simulink model "PistonDynamics"  (R2012b)
settings: Solver=ode45  StartTime=0.0  StopTime=5.0  RelTol=1e-3
undefined symbols (not defined in the file or in its folder): Ap, Ap_seal, Ar_seal, Bkp_seal, Bp1, frictionstribeck_velocity, Ka1, Lp_seal, Lr_seal, Mp1, seal_compression, seal_hardness, SealConstValue, SealType, Xp_init
settings Model: Creator=HBALLEST  LastModifiedBy=HBALLEST

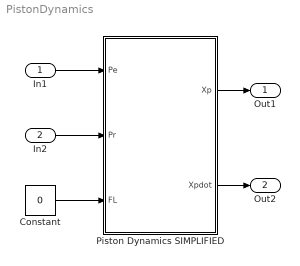
== system PistonDynamics ==
  In1 : Inport
  In2 : Inport  Port=2
  Constant : Constant  Value=0
  Piston Dynamics SIMPLIFIED : Subsystem
  Out1 : Outport
  Out2 : Outport  Port=2
  wires:
  Constant/1 -> Piston Dynamics SIMPLIFIED/3(FL)
  Piston Dynamics SIMPLIFIED/1(Xp) -> Out1/1
  Piston Dynamics SIMPLIFIED/2(Xpdot) -> Out2/1
  In2/1 -> Piston Dynamics SIMPLIFIED/2(Pr)
  In1/1 -> Piston Dynamics SIMPLIFIED/1(Pe)

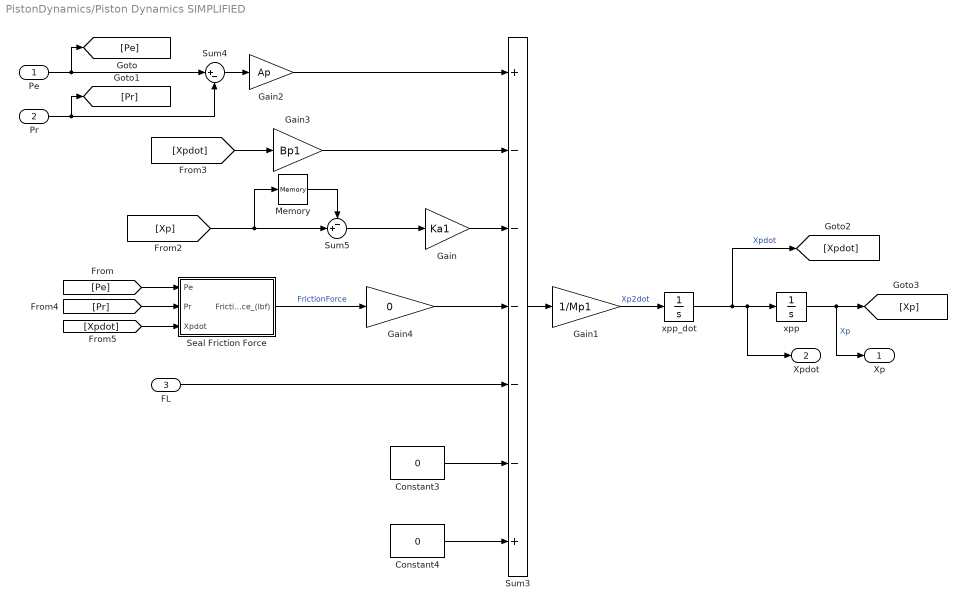
== system PistonDynamics/Piston Dynamics SIMPLIFIED ==
  Pe : Inport
  Pr : Inport  Port=2
  FL : Inport  Port=3
  Constant3 : Constant  Value=0
  Constant4 : Constant  Value=0
  Gain : Gain  Gain=Ka1
  Gain1 : Gain  Gain=1/Mp1
  Gain2 : Gain  Gain=Ap
  Gain3 : Gain  Gain=Bp1
  Gain4 : Gain  Gain=0
  Memory : Memory
  Seal Friction Force : Subsystem
  Sum3 : Sum  Inputs=+-----+
  Sum4 : Sum  Inputs=|+-
  Sum5 : Sum  Inputs=-+|
  xpp : Integrator  InitialCondition=Xp_init
  xpp_dot : Integrator
  Xp : Outport
  Xpdot : Outport  Port=2
  wires:
  Sum3/1 -> Gain1/1
  Gain1/1 -> xpp_dot/1  "Xp2dot"
  xpp_dot/1 -> xpp/1, Xpdot/1, [Xpdot]  "Xpdot"
  xpp/1 -> [Xp], Xp/1  "Xp"
  Pe/1 -> [Pe], Sum4/1
  Sum4/1 -> Gain2/1
  Gain2/1 -> Sum3/1
  [Xpdot] -> Gain3/1
  Gain3/1 -> Sum3/2
  Gain/1 -> Sum3/3
  FL/1 -> Sum3/5
  Pr/1 -> [Pr], Sum4/2
  Constant3/1 -> Sum3/6
  Constant4/1 -> Sum3/7
  Seal Friction Force/1(FrictionForce_(lbf)) -> Gain4/1  "FrictionForce"
  [Pr] -> Seal Friction Force/2(Pr)
  [Pe] -> Seal Friction Force/1(Pe)
  [Xpdot] -> Seal Friction Force/3(Xpdot)
  Sum5/1 -> Gain/1
  [Xp] -> Memory/1, Sum5/2
  Gain4/1 -> Sum3/4
  Memory/1 -> Sum5/1

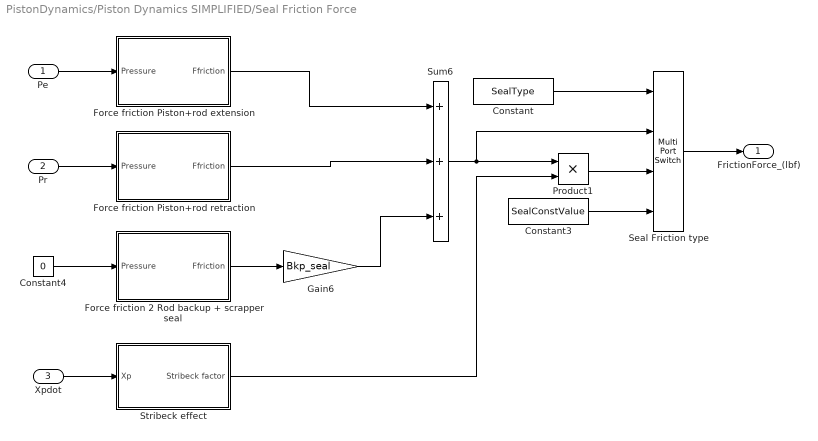
== system PistonDynamics/Piston Dynamics SIMPLIFIED/Seal Friction Force ==
  Pe : Inport
  Pr : Inport  Port=2
  Xpdot : Inport  Port=3
  Constant : Constant  Value=SealType
  Constant3 : Constant  Value=SealConstValue
  Constant4 : Constant  Value=0
  Force friction 2 Rod backup + scrapper seal : Subsystem
  Force friction Piston+rod extension : Subsystem
  Force friction Piston+rod retraction : Subsystem
  Gain6 : Gain  Gain=Bkp_seal
  Product1 : Product  RndMeth=Zero
  Seal Friction type : MultiPortSwitch
  Stribeck effect : Subsystem
  Sum6 : Sum  Inputs=+++
  FrictionForce_(lbf) : Outport
  wires:
  Constant4/1 -> Force friction 2 Rod backup + scrapper seal/1(Pressure)
  Force friction Piston+rod extension/1(Ffriction) -> Sum6/1
  Force friction Piston+rod retraction/1(Ffriction) -> Sum6/2
  Force friction 2 Rod backup + scrapper seal/1(Ffriction) -> Gain6/1
  Gain6/1 -> Sum6/3
  Pe/1 -> Force friction Piston+rod extension/1(Pressure)
  Pr/1 -> Force friction Piston+rod retraction/1(Pressure)
  Product1/1 -> Seal Friction type/3
  Sum6/1 -> Product1/1, Seal Friction type/2
  Constant/1 -> Seal Friction type/1
  Seal Friction type/1 -> FrictionForce_(lbf)/1
  Constant3/1 -> Seal Friction type/4
  Xpdot/1 -> Stribeck effect/1(Xp)
  Stribeck effect/1(Stribeck factor) -> Product1/2

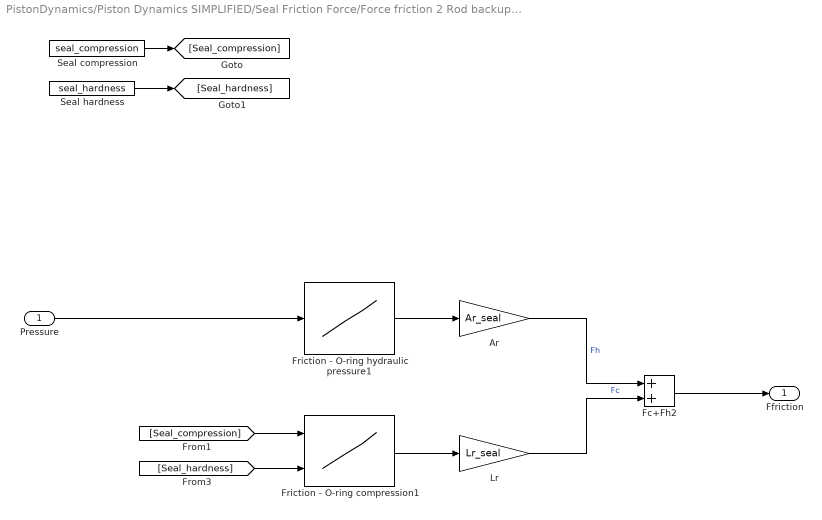
== system PistonDynamics/Piston Dynamics SIMPLIFIED/Seal Friction Force/Force friction 2 Rod backup + scrapper seal ==
  Pressure : Inport
  Ar : Gain  Gain=Ar_seal
  Fc+Fh2 : Sum
  Friction - O-ring compression1 : Lookup_n-D  BreakpointsForDimension1=[0,5,10,15,20,25]  BreakpointsForDimension2=[70,80,90]  IndexSearchMethod=Linear search  Table=reshape([0,0.3,0.65,0.97313,1.37,1.7,0,0.6,1.22,1.82,2.45,3.05,0,0.8,1.6,2.37,3.2,3.98],6,3)  RndMeth=Simplest  InputSameDT=on
  Friction - O-ring hydraulic pressure1 : Lookup_n-D  NumberOfTableDimensions=1  BreakpointsForDimension1=|  BreakpointsForDimension2=[70,80,90]  IndexSearchMethod=Linear search  Table=|  RndMeth=Simplest  InputSameDT=on
      BreakpointsForDimension1=|
      | [0
      | 500
      | 1000
      | 1500
      | 2000
      | 2500
      | 3000]
      Table=|
      | [0
      | 24.5
      | 37.5
      | 48
      | 58
      | 67
      | 72.1]
  Lr : Gain  Gain=Lr_seal
  Seal compression : Constant  Value=seal_compression
  Seal hardness : Constant  Value=seal_hardness
  Ffriction : Outport
  wires:
  Friction - O-ring compression1/1 -> Lr/1
  Lr/1 -> Fc+Fh2/2  "Fc"
  Pressure/1 -> Friction - O-ring hydraulic pressure1/1
  Friction - O-ring hydraulic pressure1/1 -> Ar/1
  Ar/1 -> Fc+Fh2/1  "Fh"
  Fc+Fh2/1 -> Ffriction/1
  Seal compression/1 -> [Seal_compression]
  [Seal_compression] -> Friction - O-ring compression1/1
  Seal hardness/1 -> [Seal_hardness]
  [Seal_hardness] -> Friction - O-ring compression1/2

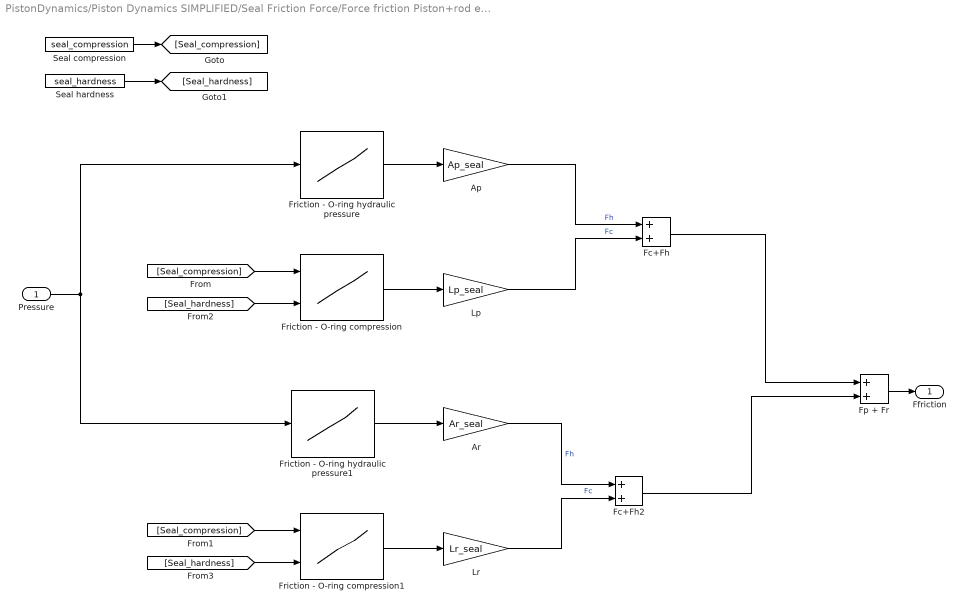
== system PistonDynamics/Piston Dynamics SIMPLIFIED/Seal Friction Force/Force friction Piston+rod extension ==
  Pressure : Inport
  Ap : Gain  Gain=Ap_seal
  Ar : Gain  Gain=Ar_seal
  Fc+Fh : Sum
  Fc+Fh2 : Sum
  Fp + Fr : Sum
  Friction - O-ring compression : Lookup_n-D  BreakpointsForDimension1=[0,5,10,15,20,25]  BreakpointsForDimension2=[70,80,90]  IndexSearchMethod=Linear search  Table=reshape([0,0.3,0.65,0.97313,1.37,1.7,0,0.6,1.22,1.82,2.45,3.05,0,0.8,1.6,2.37,3.2,3.98],6,3)  RndMeth=Simplest  InputSameDT=on
  Friction - O-ring compression1 : Lookup_n-D  BreakpointsForDimension1=[0,5,10,15,20,25]  BreakpointsForDimension2=[70,80,90]  IndexSearchMethod=Linear search  Table=reshape([0,0.3,0.65,0.97313,1.37,1.7,0,0.6,1.22,1.82,2.45,3.05,0,0.8,1.6,2.37,3.2,3.98],6,3)  RndMeth=Simplest  InputSameDT=on
  Friction - O-ring hydraulic pressure : Lookup_n-D  NumberOfTableDimensions=1  BreakpointsForDimension1=|  BreakpointsForDimension2=[70,80,90]  IndexSearchMethod=Linear search  Table=|  RndMeth=Simplest  InputSameDT=on
      BreakpointsForDimension1=|
      | [0
      | 500
      | 1000
      | 1500
      | 2000
      | 2500
      | 3000]
      Table=|
      | [0
      | 24.5
      | 37.5
      | 48
      | 58
      | 67
      | 72.1]
  Friction - O-ring hydraulic pressure1 : Lookup_n-D  NumberOfTableDimensions=1  BreakpointsForDimension1=|  BreakpointsForDimension2=[70,80,90]  IndexSearchMethod=Linear search  Table=|  RndMeth=Simplest  InputSameDT=on
      BreakpointsForDimension1=|
      | [0
      | 500
      | 1000
      | 1500
      | 2000
      | 2500
      | 3000]
      Table=|
      | [0
      | 24.5
      | 37.5
      | 48
      | 58
      | 67
      | 72.1]
  Lp : Gain  Gain=Lp_seal
  Lr : Gain  Gain=Lr_seal
  Seal compression : Constant  Value=seal_compression
  Seal hardness : Constant  Value=seal_hardness
  Ffriction : Outport
  wires:
  Friction - O-ring compression/1 -> Lp/1
  Lp/1 -> Fc+Fh/2  "Fc"
  Friction - O-ring hydraulic pressure/1 -> Ap/1
  Ap/1 -> Fc+Fh/1  "Fh"
  Fp + Fr/1 -> Ffriction/1
  Friction - O-ring compression1/1 -> Lr/1
  Lr/1 -> Fc+Fh2/2  "Fc"
  Pressure/1 -> Friction - O-ring hydraulic pressure/1, Friction - O-ring hydraulic pressure1/1
  Friction - O-ring hydraulic pressure1/1 -> Ar/1
  Ar/1 -> Fc+Fh2/1  "Fh"
  Fc+Fh2/1 -> Fp + Fr/2
  Fc+Fh/1 -> Fp + Fr/1
  Seal compression/1 -> [Seal_compression]
  [Seal_compression] -> Friction - O-ring compression/1
  [Seal_compression] -> Friction - O-ring compression1/1
  Seal hardness/1 -> [Seal_hardness]
  [Seal_hardness] -> Friction - O-ring compression/2
  [Seal_hardness] -> Friction - O-ring compression1/2

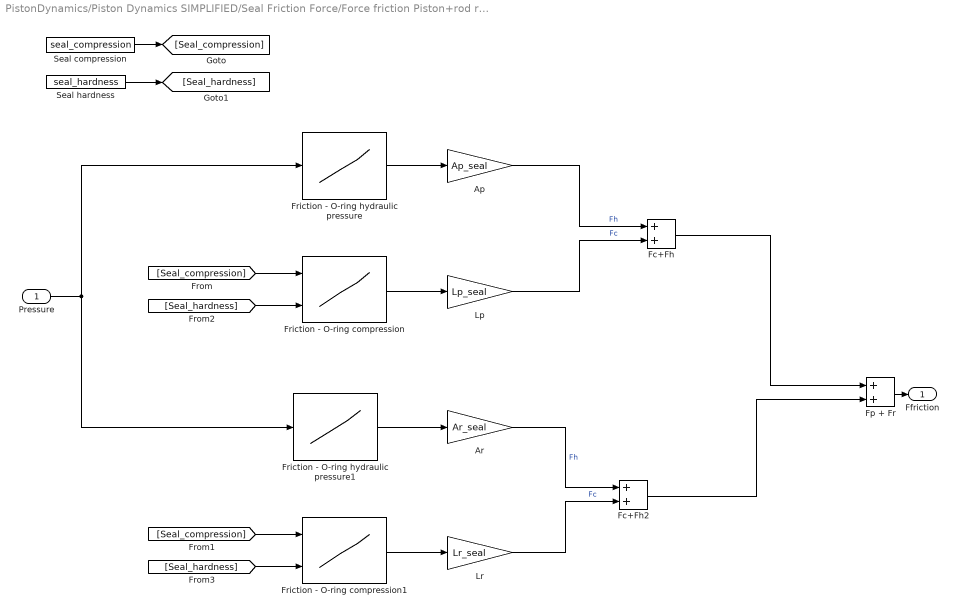
== system PistonDynamics/Piston Dynamics SIMPLIFIED/Seal Friction Force/Force friction Piston+rod retraction ==
  Pressure : Inport
  Ap : Gain  Gain=Ap_seal
  Ar : Gain  Gain=Ar_seal
  Fc+Fh : Sum
  Fc+Fh2 : Sum
  Fp + Fr : Sum
  Friction - O-ring compression : Lookup_n-D  BreakpointsForDimension1=[0,5,10,15,20,25]  BreakpointsForDimension2=[70,80,90]  IndexSearchMethod=Linear search  Table=reshape([0,0.3,0.65,0.97313,1.37,1.7,0,0.6,1.22,1.82,2.45,3.05,0,0.8,1.6,2.37,3.2,3.98],6,3)  RndMeth=Simplest  InputSameDT=on
  Friction - O-ring compression1 : Lookup_n-D  BreakpointsForDimension1=[0,5,10,15,20,25]  BreakpointsForDimension2=[70,80,90]  IndexSearchMethod=Linear search  Table=reshape([0,0.3,0.65,0.97313,1.37,1.7,0,0.6,1.22,1.82,2.45,3.05,0,0.8,1.6,2.37,3.2,3.98],6,3)  RndMeth=Simplest  InputSameDT=on
  Friction - O-ring hydraulic pressure : Lookup_n-D  NumberOfTableDimensions=1  BreakpointsForDimension1=|  BreakpointsForDimension2=[70,80,90]  IndexSearchMethod=Linear search  Table=|  RndMeth=Simplest  InputSameDT=on
      BreakpointsForDimension1=|
      | [0
      | 500
      | 1000
      | 1500
      | 2000
      | 2500
      | 3000]
      Table=|
      | [0
      | 24.5
      | 37.5
      | 48
      | 58
      | 67
      | 72.1]
  Friction - O-ring hydraulic pressure1 : Lookup_n-D  NumberOfTableDimensions=1  BreakpointsForDimension1=|  BreakpointsForDimension2=[70,80,90]  IndexSearchMethod=Linear search  Table=|  RndMeth=Simplest  InputSameDT=on
      BreakpointsForDimension1=|
      | [0
      | 500
      | 1000
      | 1500
      | 2000
      | 2500
      | 3000]
      Table=|
      | [0
      | 24.5
      | 37.5
      | 48
      | 58
      | 67
      | 72.1]
  Lp : Gain  Gain=Lp_seal
  Lr : Gain  Gain=Lr_seal
  Seal compression : Constant  Value=seal_compression
  Seal hardness : Constant  Value=seal_hardness
  Ffriction : Outport
  wires:
  Friction - O-ring compression/1 -> Lp/1
  Lp/1 -> Fc+Fh/2  "Fc"
  Friction - O-ring hydraulic pressure/1 -> Ap/1
  Ap/1 -> Fc+Fh/1  "Fh"
  Fp + Fr/1 -> Ffriction/1
  Friction - O-ring compression1/1 -> Lr/1
  Lr/1 -> Fc+Fh2/2  "Fc"
  Pressure/1 -> Friction - O-ring hydraulic pressure/1, Friction - O-ring hydraulic pressure1/1
  Friction - O-ring hydraulic pressure1/1 -> Ar/1
  Ar/1 -> Fc+Fh2/1  "Fh"
  Fc+Fh2/1 -> Fp + Fr/2
  Fc+Fh/1 -> Fp + Fr/1
  Seal compression/1 -> [Seal_compression]
  [Seal_compression] -> Friction - O-ring compression/1
  [Seal_compression] -> Friction - O-ring compression1/1
  Seal hardness/1 -> [Seal_hardness]
  [Seal_hardness] -> Friction - O-ring compression/2
  [Seal_hardness] -> Friction - O-ring compression1/2

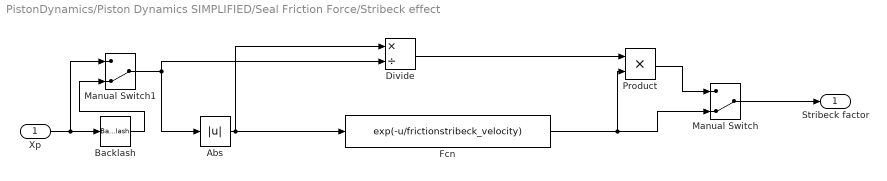
== system PistonDynamics/Piston Dynamics SIMPLIFIED/Seal Friction Force/Stribeck effect ==
  Xp : Inport
  Abs : Abs
  Backlash : Backlash  BacklashWidth=.1
  Divide : Product  Inputs=*/
  Fcn : Fcn  Expr=exp(-u/frictionstribeck_velocity)
  Manual Switch : ManualSwitch  CurrentSetting=0
  Manual Switch1 : ManualSwitch  CurrentSetting=0
  Product : Product  RndMeth=Zero
  Stribeck factor : Outport
  wires:
  Xp/1 -> Manual Switch1/1, Backlash/1
  Abs/1 -> Divide/1, Fcn/1
  Fcn/1 -> Manual Switch/2, Product/2
  Divide/1 -> Product/1
  Product/1 -> Manual Switch/1
  Manual Switch/1 -> Stribeck factor/1
  Manual Switch1/1 -> Divide/2, Abs/1
  Backlash/1 -> Manual Switch1/2
